simulink model "sampleModel7126_pp_1_1"  (R2018a)
settings: Solver=VariableStepAuto  StartTime=0.0  StopTime=10.0  RelTol=1e-3
undefined symbols (not defined in the file): DiscIntNeverNeededParam
libraries: simulink x367
(part 9 of 12)

== system sampleModel7126_pp_1_1/cfblk275/cfblk10 ==
  cfblk1 : Inport
  Action Port : ActionPort  ActionType=then
  cfblk10 : simulink/Continuous/PID Controller  Controller=PID  TimeDomain=Discrete-time  SampleTime=-1  IntegratorMethod=Forward Euler  FilterMethod=Forward Euler  Form=Parallel  UseFilter=on  ControllerParametersSource=internal  P=1  I=1  D=0  N=100  InitialConditionSource=internal  InitialConditionForIntegrator=0  InitialConditionForFilter=0  ExternalReset=none  LimitOutput=off  UpperSaturationLimit=inf  LowerSaturationLimit=-inf  LinearizeAsGain=off  AntiWindupMode=none  Kb=1  TrackingMode=off  Kt=1  PParamMin=[]  PParamMax=[]  IParamMin=[]  IParamMax=[]  DParamMin=[]  DParamMax=[]  NParamMin=[]  NParamMax=[]  KbParamMin=[]  KbParamMax=[]  KtParamMin=[]  KtParamMax=[]  POutMin=[]  POutMax=[]  IOutMin=[]  IOutMax=[]  DOutMin=[]  DOutMax=[]  NOutMin=[]  NOutMax=[]  KbOutMin=[]  KbOutMax=[]  KtOutMin=[]  KtOutMax=[]  IntegratorOutMin=[]  IntegratorOutMax=[]  FilterOutMin=[]  FilterOutMax=[]  SumOutMin=[]  SumOutMax=[]  SumI1OutMin=[]  SumI1OutMax=[]  SumI2OutMin=[]  SumI2OutMax=[]  SumI3OutMin=[]  SumI3OutMax=[]  SumDOutMin=[]  SumDOutMax=[]  SaturationOutMin=[]  SaturationOutMax=[]  IntegratorContinuousStateAttributes=''  IntegratorStateMustResolveToSignalObject=off  IntegratorRTWStateStorageClass=Auto  FilterContinuousStateAttributes=''  FilterStateMustResolveToSignalObject=off  FilterRTWStateStorageClass=Auto  DifferentiatorICPrevScaledInput=0  DifferentiatorOutMin=[]  DifferentiatorOutMax=[]  FilterDiffOutCoefMin=[]  FilterDiffOutCoefMax=[]  SumDenOutMin=[]  SumDenOutMax=[]  SumNumOutMin=[]  SumNumOutMax=[]  ReciprocalOutMin=[]  ReciprocalOutMax=[]  DivideOutMin=[]  DivideOutMax=[]  TunerSelectOption=Transfer Function Based (PID Tuner App)
  cfblk11 : DiscreteFilter
  cfblk12 : Delay  ShowEnablePort=on
      settings: InputPortMap=u0,e6
  cfblk13 : Delay
  cfblk3 : Subsystem  TreatAsAtomicUnit=on
  cfblk4 : Subsystem  TreatAsAtomicUnit=on
  cfblk5 : Subsystem  TreatAsAtomicUnit=on
  cfblk6 : DiscreteFilter
  cfblk7 : DiscreteFilter
  cfblk8 : Subsystem  TreatAsAtomicUnit=on
  cfblk9 : simulink/Discrete/Difference  ICPrevInput=0.0  OutMin=[]  OutMax=[]  OutDataTypeStr=double  OutputDataTypeScalingMode=double  OutDataType=fixdt(1, 16)  OutScaling=2^-10  DoSatur=off
  cyemi_{765..776} (12 alike) : DataTypeConversion  OutDataTypeStr=double
  emi_1205 : Subsystem  TreatAsAtomicUnit=on
  emi_{128,1207,1700,1939} (4 alike) : If  IfExpression=Inf <= u1  SampleTime=[1 0]
  emi_{129,1208,1701,1940} (4 alike) : DataTypeConversion  OutDataTypeStr=double
  emi_126 : Subsystem  TreatAsAtomicUnit=on
  emi_1698 : Subsystem  TreatAsAtomicUnit=on
  emi_1937 : Subsystem  TreatAsAtomicUnit=on
  cfblk2 : Outport
  wires:
  cfblk7/1 -> cfblk2/1, emi_1940/1
  cfblk11/1 -> cyemi_771/1, cyemi_775/1
  cyemi_765/1 -> cfblk10/1
  cfblk9/1 -> cyemi_765/1
  cyemi_766/1 -> cfblk11/1
  cfblk1/1 -> cyemi_766/1
  cyemi_767/1 -> cfblk12/1
  cfblk10/1 -> cyemi_767/1
  cyemi_768/1 -> cfblk12/2
  cfblk13/1 -> cyemi_768/1
  cyemi_769/1 -> cfblk13/1
  cfblk12/1 -> cyemi_772/1, emi_129/1
  cyemi_773/1 -> cfblk6/1
  cyemi_774/1 -> cfblk7/1
  cfblk6/1 -> cyemi_774/1, emi_1701/1
  cyemi_776/1 -> cfblk9/1
  cyemi_772/1 -> cfblk5/1(emi_124)
  cfblk5/1(emi_125) -> cyemi_769/1
  emi_128/1 -> cfblk5/Action
  emi_128/2 -> emi_126/Action
  emi_129/1 -> emi_128/1
  cyemi_775/1 -> cfblk8/1(emi_1203)
  cfblk8/1(emi_1204) -> cyemi_773/1
  emi_1207/1 -> cfblk8/Action
  emi_1207/2 -> emi_1205/Action
  emi_1208/1 -> emi_1207/1
  cyemi_770/1 -> cfblk3/1(emi_1696)
  cfblk3/1(emi_1697) -> emi_1208/1, cyemi_776/1
  emi_1700/1 -> cfblk3/Action
  emi_1700/2 -> emi_1698/Action
  emi_1701/1 -> emi_1700/1
  cyemi_771/1 -> cfblk4/1(emi_1935)
  cfblk4/1(emi_1936) -> cyemi_770/1
  emi_1939/1 -> cfblk4/Action
  emi_1939/2 -> emi_1937/Action
  emi_1940/1 -> emi_1939/1

== system sampleModel7126_pp_1_1/cfblk275/cfblk11 ==
  cfblk1 : Inport
  Action Port : ActionPort  ActionType=else
  cfblk10 : simulink/Discrete/Transfer Fcn Real Zero  ZeroZ=0.75  ICPrevInput=0.0  DoSatur=off
      settings: SourceProductName=Simulink  SourceProductBaseCode=SL
  cfblk11 : Subsystem  TreatAsAtomicUnit=on
  cfblk12 : DiscreteIntegrator  SampleTime=-1  OutDataTypeStr=double  ICPrevOutput=DiscIntNeverNeededParam  ICPrevScaledInput=DiscIntNeverNeededParam
  cfblk13 : DiscreteZeroPole  Poles=[0 0.5]  Gain=1  SampleTime=-1
  cfblk14 : Subsystem  TreatAsAtomicUnit=on
  cfblk18 : Delay
  cfblk3 : Subsystem  TreatAsAtomicUnit=on
  cfblk4 : simulink/Continuous/PID Controller  Controller=PID  TimeDomain=Discrete-time  SampleTime=-1  IntegratorMethod=Forward Euler  FilterMethod=Forward Euler  Form=Parallel  UseFilter=on  ControllerParametersSource=internal  P=1  I=1  D=0  N=100  InitialConditionSource=internal  InitialConditionForIntegrator=0  InitialConditionForFilter=0  ExternalReset=none  LimitOutput=off  UpperSaturationLimit=inf  LowerSaturationLimit=-inf  LinearizeAsGain=off  AntiWindupMode=none  Kb=1  TrackingMode=off  Kt=1  PParamMin=[]  PParamMax=[]  IParamMin=[]  IParamMax=[]  DParamMin=[]  DParamMax=[]  NParamMin=[]  NParamMax=[]  KbParamMin=[]  KbParamMax=[]  KtParamMin=[]  KtParamMax=[]  POutMin=[]  POutMax=[]  IOutMin=[]  IOutMax=[]  DOutMin=[]  DOutMax=[]  NOutMin=[]  NOutMax=[]  KbOutMin=[]  KbOutMax=[]  KtOutMin=[]  KtOutMax=[]  IntegratorOutMin=[]  IntegratorOutMax=[]  FilterOutMin=[]  FilterOutMax=[]  SumOutMin=[]  SumOutMax=[]  SumI1OutMin=[]  SumI1OutMax=[]  SumI2OutMin=[]  SumI2OutMax=[]  SumI3OutMin=[]  SumI3OutMax=[]  SumDOutMin=[]  SumDOutMax=[]  SaturationOutMin=[]  SaturationOutMax=[]  IntegratorContinuousStateAttributes=''  IntegratorStateMustResolveToSignalObject=off  IntegratorRTWStateStorageClass=Auto  FilterContinuousStateAttributes=''  FilterStateMustResolveToSignalObject=off  FilterRTWStateStorageClass=Auto  DifferentiatorICPrevScaledInput=0  DifferentiatorOutMin=[]  DifferentiatorOutMax=[]  FilterDiffOutCoefMin=[]  FilterDiffOutCoefMax=[]  SumDenOutMin=[]  SumDenOutMax=[]  SumNumOutMin=[]  SumNumOutMax=[]  ReciprocalOutMin=[]  ReciprocalOutMax=[]  DivideOutMin=[]  DivideOutMax=[]  TunerSelectOption=Transfer Function Based (PID Tuner App)
  cfblk5 : DiscreteZeroPole  Poles=[0 0.5]  Gain=1  SampleTime=-1
  cfblk6 : DiscreteStateSpace  SampleTime=-1
  cfblk7 : Delay  ShowEnablePort=on
      settings: InputPortMap=u0,e6
  cfblk8 : UnitDelay  SampleTime=-1
  cfblk9 : Subsystem  TreatAsAtomicUnit=on
  cyemi_{778..791} (14 alike) : DataTypeConversion  OutDataTypeStr=double
  emi_1322 : Subsystem  TreatAsAtomicUnit=on
  emi_{567,609,1324,2191} (4 alike) : If  IfExpression=0 <= u1  SampleTime=[1 0]
  emi_{568,610,1325,2192} (4 alike) : DataTypeConversion  OutDataTypeStr=double
  emi_2189 : Subsystem  TreatAsAtomicUnit=on
  emi_565 : Subsystem  TreatAsAtomicUnit=on
  emi_607 : Subsystem  TreatAsAtomicUnit=on
  cfblk2 : Outport
  cfblk15 : Outport  Port=2
  cfblk16 : Outport  Port=3
  cfblk17 : Outport  Port=4
  wires:
  cfblk5/1 -> cyemi_779/1, cyemi_780/1, emi_610/1
  cfblk8/1 -> cfblk15/1
  cfblk10/1 -> cfblk16/1, cyemi_784/1
  cfblk6/1 -> cfblk17/1, cyemi_790/1
  cyemi_778/1 -> cfblk10/1
  cfblk7/1 -> cyemi_778/1
  cyemi_780/1 -> cfblk12/1
  cyemi_781/1 -> cfblk13/1
  cfblk4/1 -> cyemi_782/1
  cyemi_783/1 -> cfblk18/1
  cyemi_785/1 -> cfblk4/1
  cfblk13/1 -> cyemi_785/1
  cyemi_786/1 -> cfblk5/1
  cfblk18/1 -> cyemi_786/1, emi_1325/1
  cyemi_787/1 -> cfblk6/1
  cyemi_788/1 -> cfblk7/1
  cfblk1/1 -> cyemi_788/1
  cyemi_789/1 -> cfblk7/2
  cfblk12/1 -> cyemi_789/1, emi_2192/1
  cyemi_790/1 -> cfblk8/1
  cyemi_782/1 -> cfblk14/1(emi_563)
  cfblk14/1(emi_564) -> cfblk2/1
  emi_567/1 -> cfblk14/Action
  emi_567/2 -> emi_565/Action
  emi_568/1 -> emi_567/1
  cyemi_784/1 -> cfblk3/1(emi_605)
  cfblk3/1(emi_606) -> cyemi_787/1
  emi_609/1 -> cfblk3/Action
  emi_609/2 -> emi_607/Action
  emi_610/1 -> emi_609/1
  cyemi_791/1 -> cfblk9/1(emi_1320)
  cfblk9/1(emi_1321) -> cyemi_783/1
  emi_1324/1 -> cfblk9/Action
  emi_1324/2 -> emi_1322/Action
  emi_1325/1 -> emi_1324/1
  cyemi_779/1 -> cfblk11/1(emi_2187)
  cfblk11/1(emi_2188) -> emi_568/1, cyemi_791/1, cyemi_781/1
  emi_2191/1 -> cfblk11/Action
  emi_2191/2 -> emi_2189/Action
  emi_2192/1 -> emi_2191/1

== system sampleModel7126_pp_1_1/cfblk276/cfblk14 ==
  emi_1820 : Inport
  Action Port : ActionPort  ActionType=then
  cfblk14 : Delay
  emi_1821 : Outport
  wires:
  emi_1820/1 -> cfblk14/1
  cfblk14/1 -> emi_1821/1

== system sampleModel7126_pp_1_1/cfblk276/cfblk3 ==
  emi_238 : Inport
  Action Port : ActionPort  ActionType=then
  cfblk3 : simulink/Discrete/Transfer Fcn First Order  PoleZ=0.95  ICPrevOutput=0.0  DoSatur=off
      settings: SourceProductName=Simulink
  emi_239 : Outport
  wires:
  emi_238/1 -> cfblk3/1
  cfblk3/1 -> emi_239/1

== system sampleModel7126_pp_1_1/cfblk276/cfblk4 ==
  emi_79 : Inport
  Action Port : ActionPort  ActionType=then
  cfblk4 : UnitDelay  SampleTime=-1
  emi_80 : Outport
  wires:
  emi_79/1 -> cfblk4/1
  cfblk4/1 -> emi_80/1

== system sampleModel7126_pp_1_1/cfblk276/cfblk5 ==
  emi_767 : Inport
  Action Port : ActionPort  ActionType=then
  cfblk5 : DiscreteZeroPole  Poles=[0 0.5]  Gain=1  SampleTime=-1
  emi_768 : Outport
  wires:
  emi_767/1 -> cfblk5/1
  cfblk5/1 -> emi_768/1

== system sampleModel7126_pp_1_1/cfblk276/cfblk6 ==
  emi_1102 : Inport
  emi_1103 : Inport  Port=2
  Action Port : ActionPort  ActionType=then
  cfblk6 : Delay  ShowEnablePort=on
      settings: InputPortMap=u0,e6
  emi_1104 : Outport
  wires:
  emi_1102/1 -> cfblk6/1
  emi_1103/1 -> cfblk6/2
  cfblk6/1 -> emi_1104/1

== system sampleModel7126_pp_1_1/cfblk276/cfblk7 ==
  emi_1355 : Inport
  Action Port : ActionPort  ActionType=then
  cfblk7 : Delay
  emi_1356 : Outport
  wires:
  emi_1355/1 -> cfblk7/1
  cfblk7/1 -> emi_1356/1

== system sampleModel7126_pp_1_1/cfblk276/emi_1105 ==
  Action Port : ActionPort  ActionType=else
  emi_1106 : Assertion

== system sampleModel7126_pp_1_1/cfblk276/emi_1357 ==
  Action Port : ActionPort  ActionType=else
  emi_1358 : Assertion

== system sampleModel7126_pp_1_1/cfblk276/emi_1822 ==
  Action Port : ActionPort  ActionType=else
  emi_1823 : Assertion

== system sampleModel7126_pp_1_1/cfblk276/emi_240 ==
  Action Port : ActionPort  ActionType=else
  emi_241 : Assertion

== system sampleModel7126_pp_1_1/cfblk276/emi_769 ==
  Action Port : ActionPort  ActionType=else
  emi_770 : Assertion

== system sampleModel7126_pp_1_1/cfblk276/emi_81 ==
  Action Port : ActionPort  ActionType=else
  emi_82 : Assertion

== system sampleModel7126_pp_1_1/cfblk277/cfblk11 ==
  emi_746 : Inport
  Action Port : ActionPort  ActionType=then
  cfblk11 : Delay
  emi_747 : Outport
  wires:
  emi_746/1 -> cfblk11/1
  cfblk11/1 -> emi_747/1

== system sampleModel7126_pp_1_1/cfblk277/cfblk13 ==
  emi_1639 : Inport
  Action Port : ActionPort  ActionType=then
  cfblk13 : simulink/Discrete/Transfer Fcn Lead or Lag  PoleZ=0.95  ZeroZ=0.75  ICPrevOutput=0.0  ICPrevInput=0.0  DoSatur=off
      settings: SourceProductName=Simulink  SourceProductBaseCode=SL
  emi_1640 : Outport
  wires:
  emi_1639/1 -> cfblk13/1
  cfblk13/1 -> emi_1640/1

== system sampleModel7126_pp_1_1/cfblk277/cfblk18 ==
  cfblk1 : Inport
  cfblk8 : Inport  Port=2
  Action Port : ActionPort  ActionType=then
  cfblk3 : Subsystem  TreatAsAtomicUnit=on
  cfblk4 : DiscreteFir
  cfblk5 : Subsystem  TreatAsAtomicUnit=on
  cfblk6 : DiscreteZeroPole  Poles=[0 0.5]  Gain=1  SampleTime=-1
  cfblk7 : Subsystem  TreatAsAtomicUnit=on
  cfblk9 : Delay
  cyemi_{823..829} (7 alike) : DataTypeConversion  OutDataTypeStr=double
  emi_2154 : Subsystem  TreatAsAtomicUnit=on
  emi_2156 : If  IfExpression=Inf <= u1  SampleTime=[1 0]
  emi_2157 : DataTypeConversion  OutDataTypeStr=double
  emi_551 : Subsystem  TreatAsAtomicUnit=on
  emi_553 : If  IfExpression=Inf <= u1
  emi_554 : DataTypeConversion  OutDataTypeStr=double
  emi_940 : Subsystem  TreatAsAtomicUnit=on
  emi_942 : If  IfExpression=Inf <= u1  SampleTime=[1 0]
  emi_943 : DataTypeConversion  OutDataTypeStr=double
  cfblk2 : Outport
  wires:
  cfblk6/1 -> cyemi_823/1
  cyemi_824/1 -> cfblk4/1
  cyemi_826/1 -> cfblk6/1
  cfblk8/1 -> cyemi_826/1
  cfblk9/1 -> cyemi_827/1, emi_943/1
  cfblk1/1 -> cyemi_828/1
  cyemi_829/1 -> cfblk9/1
  cfblk4/1 -> cyemi_829/1, emi_554/1, emi_2157/1
  cyemi_823/1 -> cfblk3/1(emi_549)
  cfblk3/1(emi_550) -> cfblk2/1
  emi_553/1 -> cfblk3/Action
  emi_553/2 -> emi_551/Action
  emi_554/1 -> emi_553/1
  cyemi_825/1 -> cfblk5/1(emi_938)
  cfblk5/1(emi_939) -> cyemi_824/1
  emi_942/1 -> cfblk5/Action
  emi_942/2 -> emi_940/Action
  emi_943/1 -> emi_942/1
  cyemi_827/1 -> cfblk7/1(emi_2151)
  cyemi_828/1 -> cfblk7/2(emi_2152)
  cfblk7/1(emi_2153) -> cyemi_825/1
  emi_2156/1 -> cfblk7/Action
  emi_2156/2 -> emi_2154/Action
  emi_2157/1 -> emi_2156/1

== system sampleModel7126_pp_1_1/cfblk277/cfblk19 ==
  cfblk1 : Inport
  Action Port : ActionPort  ActionType=else
  cfblk{9..12} (4 alike) : Delay
  cfblk3 : simulink/Continuous/PID Controller (2DOF)  Controller=PID  TimeDomain=Discrete-time  SampleTime=-1  IntegratorMethod=Forward Euler  FilterMethod=Forward Euler  Form=Parallel  UseFilter=on  ControllerParametersSource=internal  P=1  I=1  D=0  N=100  b=1  c=1  InitialConditionSource=internal  InitialConditionForIntegrator=0  InitialConditionForFilter=0  ExternalReset=none  LimitOutput=off  UpperSaturationLimit=inf  LowerSaturationLimit=-inf  LinearizeAsGain=off  AntiWindupMode=none  Kb=1  TrackingMode=off  Kt=1  PParamMin=[]  PParamMax=[]  IParamMin=[]  IParamMax=[]  DParamMin=[]  DParamMax=[]  NParamMin=[]  NParamMax=[]  bParamMin=[]  bParamMax=[]  cParamMin=[]  cParamMax=[]  KbParamMin=[]  KbParamMax=[]  KtParamMin=[]  KtParamMax=[]  POutMin=[]  POutMax=[]  IOutMin=[]  IOutMax=[]  DOutMin=[]  DOutMax=[]  NOutMin=[]  NOutMax=[]  bOutMin=[]  bOutMax=[]  cOutMin=[]  cOutMax=[]  KbOutMin=[]  KbOutMax=[]  KtOutMin=[]  KtOutMax=[]  IntegratorOutMin=[]  IntegratorOutMax=[]  FilterOutMin=[]  FilterOutMax=[]  SumOutMin=[]  SumOutMax=[]  Sum1OutMin=[]  Sum1OutMax=[]  Sum2OutMin=[]  Sum2OutMax=[]  Sum3OutMin=[]  Sum3OutMax=[]  SumI1OutMin=[]  SumI1OutMax=[]  SumI2OutMin=[]  SumI2OutMax=[]  SumI3OutMin=[]  SumI3OutMax=[]  SumDOutMin=[]  SumDOutMax=[]  SaturationOutMin=[]  SaturationOutMax=[]  IntegratorContinuousStateAttributes=''  IntegratorStateMustResolveToSignalObject=off  IntegratorRTWStateStorageClass=Auto  FilterContinuousStateAttributes=''  FilterStateMustResolveToSignalObject=off  FilterRTWStateStorageClass=Auto  DifferentiatorICPrevScaledInput=0  DifferentiatorOutMin=[]  DifferentiatorOutMax=[]  FilterDiffOutCoefMin=[]  FilterDiffOutCoefMax=[]  SumDenOutMin=[]  SumDenOutMax=[]  SumNumOutMin=[]  SumNumOutMax=[]  ReciprocalOutMin=[]  ReciprocalOutMax=[]  DivideOutMin=[]  DivideOutMax=[]  TunerSelectOption=Transfer Function Based (PID Tuner App)
  cfblk4 : Delay  ShowEnablePort=on
      settings: InputPortMap=u0,e6
  cfblk5 : Subsystem  TreatAsAtomicUnit=on
  cfblk6 : Subsystem  TreatAsAtomicUnit=on
  cfblk7 : Delay  ShowEnablePort=on
      settings: InputPortMap=u0,e6
  cfblk8 : Subsystem  TreatAsAtomicUnit=on
  cyemi_{831..843} (13 alike) : DataTypeConversion  OutDataTypeStr=double
  emi_1599 : Subsystem  TreatAsAtomicUnit=on
  emi_1601 : If  IfExpression=Inf <= u1  SampleTime=[1 0]
  emi_1602 : DataTypeConversion  OutDataTypeStr=double
  emi_1908 : Subsystem  TreatAsAtomicUnit=on
  emi_1910 : If  IfExpression=Inf <= u1  SampleTime=[1 0]
  emi_1911 : DataTypeConversion  OutDataTypeStr=double
  emi_381 : Subsystem  TreatAsAtomicUnit=on
  emi_383 : If  IfExpression=Inf <= u1  SampleTime=[1 0]
  emi_384 : DataTypeConversion  OutDataTypeStr=double
  cfblk2 : Outport
  wires:
  cfblk1/1 -> cfblk2/1
  cfblk4/1 -> cyemi_831/1, cyemi_843/1
  cfblk3/1 -> cyemi_836/1, cyemi_841/1
  cfblk7/1 -> cyemi_837/1, cyemi_842/1
  cyemi_831/1 -> cfblk10/1
  cyemi_832/1 -> cfblk11/1
  cyemi_833/1 -> cfblk12/1
  cyemi_834/1 -> cfblk3/1
  cfblk9/1 -> cyemi_834/1, emi_1911/1
  cyemi_835/1 -> cfblk3/2
  cfblk10/1 -> cyemi_835/1, emi_1602/1
  cyemi_836/1 -> cfblk4/1
  cyemi_837/1 -> cfblk4/2
  cfblk12/1 -> cyemi_838/1, emi_384/1
  cyemi_840/1 -> cfblk7/1
  cfblk11/1 -> cyemi_840/1
  cyemi_841/1 -> cfblk7/2
  cyemi_843/1 -> cfblk9/1
  cyemi_839/1 -> cfblk6/1(emi_379)
  cfblk6/1(emi_380) -> cyemi_833/1
  emi_383/1 -> cfblk6/Action
  emi_383/2 -> emi_381/Action
  emi_384/1 -> emi_383/1
  cyemi_842/1 -> cfblk8/1(emi_1597)
  cfblk8/1(emi_1598) -> cyemi_832/1
  emi_1601/1 -> cfblk8/Action
  emi_1601/2 -> emi_1599/Action
  emi_1602/1 -> emi_1601/1
  cyemi_838/1 -> cfblk5/1(emi_1906)
  cfblk5/1(emi_1907) -> cyemi_839/1
  emi_1910/1 -> cfblk5/Action
  emi_1910/2 -> emi_1908/Action
  emi_1911/1 -> emi_1910/1

== system sampleModel7126_pp_1_1/cfblk277/cfblk21 ==
  emi_1646 : Inport
  Action Port : ActionPort  ActionType=then
  cfblk21 : Delay
  emi_1647 : Outport
  wires:
  emi_1646/1 -> cfblk21/1
  cfblk21/1 -> emi_1647/1

== system sampleModel7126_pp_1_1/cfblk277/cfblk23 ==
  emi_2059 : Inport
  Action Port : ActionPort  ActionType=then
  cfblk23 : Delay
  emi_2060 : Outport
  wires:
  emi_2059/1 -> cfblk23/1
  cfblk23/1 -> emi_2060/1

== system sampleModel7126_pp_1_1/cfblk277/cfblk3 ==
  emi_1327 : Inport
  Action Port : ActionPort  ActionType=then
  cfblk3 : simulink/Discrete/Transfer Fcn Real Zero  ZeroZ=0.75  ICPrevInput=0.0  DoSatur=off
      settings: SourceProductName=Simulink  SourceProductBaseCode=SL
  emi_1328 : Outport
  wires:
  emi_1327/1 -> cfblk3/1
  cfblk3/1 -> emi_1328/1

== system sampleModel7126_pp_1_1/cfblk277/cfblk5 ==
  emi_2087 : Inport
  Action Port : ActionPort  ActionType=then
  cfblk5 : Delay
  emi_2088 : Outport
  wires:
  emi_2087/1 -> cfblk5/1
  cfblk5/1 -> emi_2088/1

== system sampleModel7126_pp_1_1/cfblk277/cfblk6 ==
  emi_1440 : Inport
  Action Port : ActionPort  ActionType=then
  cfblk6 : UnitDelay  SampleTime=-1
  emi_1441 : Outport
  wires:
  emi_1440/1 -> cfblk6/1
  cfblk6/1 -> emi_1441/1

== system sampleModel7126_pp_1_1/cfblk277/cfblk7 ==
  emi_626 : Inport
  Action Port : ActionPort  ActionType=then
  cfblk7 : UnitDelay  SampleTime=-1
  emi_627 : Outport
  wires:
  emi_626/1 -> cfblk7/1
  cfblk7/1 -> emi_627/1

== system sampleModel7126_pp_1_1/cfblk277/cfblk8 ==
  emi_216 : Inport
  Action Port : ActionPort  ActionType=then
  cfblk8 : DiscreteFilter
  emi_217 : Outport
  wires:
  emi_216/1 -> cfblk8/1
  cfblk8/1 -> emi_217/1

== system sampleModel7126_pp_1_1/cfblk277/emi_1329 ==
  Action Port : ActionPort  ActionType=else
  emi_1330 : Assertion

== system sampleModel7126_pp_1_1/cfblk277/emi_1442 ==
  Action Port : ActionPort  ActionType=else
  emi_1443 : Assertion

== system sampleModel7126_pp_1_1/cfblk277/emi_1641 ==
  Action Port : ActionPort  ActionType=else
  emi_1642 : Assertion

== system sampleModel7126_pp_1_1/cfblk277/emi_1648 ==
  Action Port : ActionPort  ActionType=else
  emi_1649 : Assertion

== system sampleModel7126_pp_1_1/cfblk277/emi_2061 ==
  Action Port : ActionPort  ActionType=else
  emi_2062 : Assertion

== system sampleModel7126_pp_1_1/cfblk277/emi_2089 ==
  Action Port : ActionPort  ActionType=else
  emi_2090 : Assertion

== system sampleModel7126_pp_1_1/cfblk277/emi_218 ==
  Action Port : ActionPort  ActionType=else
  emi_219 : Assertion

== system sampleModel7126_pp_1_1/cfblk277/emi_628 ==
  Action Port : ActionPort  ActionType=else
  emi_629 : Assertion

== system sampleModel7126_pp_1_1/cfblk277/emi_748 ==
  Action Port : ActionPort  ActionType=else
  emi_749 : Assertion

== system sampleModel7126_pp_1_1/cfblk278/cfblk12 ==
  cfblk1 : Inport
  Action Port : ActionPort  ActionType=then
  cfblk10 : DiscreteFir
  cfblk11 : simulink/Discrete/Transfer Fcn Lead or Lag  PoleZ=0.95  ZeroZ=0.75  ICPrevOutput=0.0  ICPrevInput=0.0  DoSatur=off
      settings: SourceProductName=Simulink  SourceProductBaseCode=SL
  cfblk12 : Subsystem  TreatAsAtomicUnit=on
  cfblk{4,13..15} (4 alike) : Delay
  cfblk3 : simulink/Discrete/Transfer Fcn Lead or Lag  PoleZ=0.95  ZeroZ=0.75  ICPrevOutput=0.0  ICPrevInput=0.0  DoSatur=off
      settings: SourceProductName=Simulink  SourceProductBaseCode=SL
  cfblk5 : simulink/Continuous/PID Controller  Controller=PID  TimeDomain=Discrete-time  SampleTime=-1  IntegratorMethod=Forward Euler  FilterMethod=Forward Euler  Form=Parallel  UseFilter=on  ControllerParametersSource=internal  P=1  I=1  D=0  N=100  InitialConditionSource=internal  InitialConditionForIntegrator=0  InitialConditionForFilter=0  ExternalReset=none  LimitOutput=off  UpperSaturationLimit=inf  LowerSaturationLimit=-inf  LinearizeAsGain=off  AntiWindupMode=none  Kb=1  TrackingMode=off  Kt=1  PParamMin=[]  PParamMax=[]  IParamMin=[]  IParamMax=[]  DParamMin=[]  DParamMax=[]  NParamMin=[]  NParamMax=[]  KbParamMin=[]  KbParamMax=[]  KtParamMin=[]  KtParamMax=[]  POutMin=[]  POutMax=[]  IOutMin=[]  IOutMax=[]  DOutMin=[]  DOutMax=[]  NOutMin=[]  NOutMax=[]  KbOutMin=[]  KbOutMax=[]  KtOutMin=[]  KtOutMax=[]  IntegratorOutMin=[]  IntegratorOutMax=[]  FilterOutMin=[]  FilterOutMax=[]  SumOutMin=[]  SumOutMax=[]  SumI1OutMin=[]  SumI1OutMax=[]  SumI2OutMin=[]  SumI2OutMax=[]  SumI3OutMin=[]  SumI3OutMax=[]  SumDOutMin=[]  SumDOutMax=[]  SaturationOutMin=[]  SaturationOutMax=[]  IntegratorContinuousStateAttributes=''  IntegratorStateMustResolveToSignalObject=off  IntegratorRTWStateStorageClass=Auto  FilterContinuousStateAttributes=''  FilterStateMustResolveToSignalObject=off  FilterRTWStateStorageClass=Auto  DifferentiatorICPrevScaledInput=0  DifferentiatorOutMin=[]  DifferentiatorOutMax=[]  FilterDiffOutCoefMin=[]  FilterDiffOutCoefMax=[]  SumDenOutMin=[]  SumDenOutMax=[]  SumNumOutMin=[]  SumNumOutMax=[]  ReciprocalOutMin=[]  ReciprocalOutMax=[]  DivideOutMin=[]  DivideOutMax=[]  TunerSelectOption=Transfer Function Based (PID Tuner App)
  cfblk6 : Subsystem  TreatAsAtomicUnit=on
  cfblk7 : DiscreteIntegrator  SampleTime=-1  OutDataTypeStr=double  ICPrevOutput=DiscIntNeverNeededParam  ICPrevScaledInput=DiscIntNeverNeededParam
  cfblk8 : simulink/Discrete/Tapped Delay  vinit=0.0  samptime=-1  NumDelays=1  DelayOrder=Oldest  includeCurrent=off
  cfblk9 : DiscreteFir
  cyemi_{859..871} (13 alike) : DataTypeConversion  OutDataTypeStr=double
  emi_2139 : Subsystem  TreatAsAtomicUnit=on
  emi_2141 : If  IfExpression=Inf <= u1  SampleTime=[1 0]
  emi_2142 : DataTypeConversion  OutDataTypeStr=double
  emi_74 : Subsystem  TreatAsAtomicUnit=on
  emi_76 : If  IfExpression=Inf <= u1  SampleTime=[1 0]
  emi_77 : DataTypeConversion  OutDataTypeStr=double
  cfblk2 : Outport
  wires:
  cfblk1/1 -> cfblk2/1
  cyemi_859/1 -> cfblk10/1
  cfblk9/1 -> cyemi_859/1, emi_2142/1
  cyemi_860/1 -> cfblk11/1
  cfblk8/1 -> cyemi_860/1
  cfblk7/1 -> cyemi_861/1
  cyemi_862/1 -> cfblk13/1
  cfblk11/1 -> cyemi_862/1
  cyemi_863/1 -> cfblk14/1
  cyemi_864/1 -> cfblk15/1
  cfblk10/1 -> cyemi_864/1
  cyemi_865/1 -> cfblk3/1
  cfblk13/1 -> cyemi_865/1
  cyemi_866/1 -> cfblk4/1
  cfblk14/1 -> cyemi_866/1
  cyemi_867/1 -> cfblk5/1
  cfblk15/1 -> cyemi_867/1
  cfblk4/1 -> cyemi_868/1
  cyemi_869/1 -> cfblk7/1
  cfblk5/1 -> cyemi_869/1
  cyemi_870/1 -> cfblk8/1
  cfblk3/1 -> cyemi_870/1
  cyemi_871/1 -> cfblk9/1
  cyemi_868/1 -> cfblk6/1(emi_72)
  cfblk6/1(emi_73) -> cyemi_863/1
  emi_76/1 -> cfblk6/Action
  emi_76/2 -> emi_74/Action
  emi_77/1 -> emi_76/1
  cyemi_861/1 -> cfblk12/1(emi_2137)
  cfblk12/1(emi_2138) -> emi_77/1, cyemi_871/1
  emi_2141/1 -> cfblk12/Action
  emi_2141/2 -> emi_2139/Action
  emi_2142/1 -> emi_2141/1

== system sampleModel7126_pp_1_1/cfblk278/cfblk13 ==
  cfblk1 : Inport
  cfblk8 : Inport  Port=2
  cfblk9 : Inport  Port=3
  Action Port : ActionPort  ActionType=else
  cfblk3 : DiscreteFir
  cfblk4 : Delay
  cfblk5 : simulink/Discrete/Transfer Fcn Real Zero  ZeroZ=0.75  ICPrevInput=0.0  DoSatur=off
      settings: SourceProductName=Simulink  SourceProductBaseCode=SL
  cfblk6 : DiscreteTransferFcn
  cfblk7 : DiscreteIntegrator  SampleTime=-1  OutDataTypeStr=double  ICPrevOutput=DiscIntNeverNeededParam  ICPrevScaledInput=DiscIntNeverNeededParam
  cyemi_{875..879} (5 alike) : DataTypeConversion  OutDataTypeStr=double
  cfblk2 : Outport
  wires:
  cfblk9/1 -> cfblk2/1
  cyemi_875/1 -> cfblk3/1
  cfblk1/1 -> cyemi_875/1
  cyemi_876/1 -> cfblk4/1
  cfblk3/1 -> cyemi_876/1
  cyemi_877/1 -> cfblk5/1
  cfblk7/1 -> cyemi_877/1
  cyemi_878/1 -> cfblk6/1
  cfblk5/1 -> cyemi_878/1
  cyemi_879/1 -> cfblk7/1
  cfblk8/1 -> cyemi_879/1

== system sampleModel7126_pp_1_1/cfblk278/cfblk14 ==
  cfblk1 : Inport
  cfblk9 : Inport  Port=2
  cfblk10 : Inport  Port=3
  cfblk11 : Inport  Port=4
  cfblk12 : Inport  Port=5
  cfblk13 : Inport  Port=6
  cfblk14 : Inport  Port=7
  cfblk15 : Inport  Port=8
  Action Port : ActionPort  ActionType=then
  cfblk17 : Delay
  cfblk3 : DiscreteFilter
  cfblk4 : Delay  DelayLengthSource=Input port
      settings: InputPortMap=u0,p1
  cfblk5 : DiscreteTransferFcn
  cfblk6 : Delay  DelayLengthSource=Input port
      settings: InputPortMap=u0,p1
  cfblk7 : DiscreteStateSpace  SampleTime=-1
  cfblk8 : UnitDelay  SampleTime=-1
  cyemi_{888..896} (9 alike) : DataTypeConversion  OutDataTypeStr=double
  cfblk2 : Outport
  cfblk16 : Outport  Port=2
  wires:
  cfblk11/1 -> cfblk16/1
  cfblk7/1 -> cfblk2/1
  cyemi_888/1 -> cfblk17/1
  cfblk8/1 -> cyemi_888/1
  cyemi_889/1 -> cfblk3/1
  cfblk5/1 -> cyemi_889/1
  cyemi_890/1 -> cfblk4/1
  cfblk9/1 -> cyemi_890/1
  cyemi_891/1 -> cfblk4/2
  cfblk1/1 -> cyemi_891/1
  cyemi_892/1 -> cfblk5/1
  cfblk15/1 -> cyemi_892/1
  cyemi_893/1 -> cfblk6/1
  cfblk3/1 -> cyemi_893/1
  cyemi_894/1 -> cfblk6/2
  cfblk17/1 -> cyemi_894/1
  cyemi_895/1 -> cfblk7/1
  cfblk12/1 -> cyemi_895/1
  cyemi_896/1 -> cfblk8/1
  cfblk6/1 -> cyemi_896/1

== system sampleModel7126_pp_1_1/cfblk278/cfblk15 ==
  cfblk1 : Inport
  cfblk13 : Inport  Port=2
  cfblk14 : Inport  Port=3
  cfblk15 : Inport  Port=4
  Action Port : ActionPort  ActionType=else
  cfblk10 : simulink/Discrete/Tapped Delay  vinit=0.0  samptime=-1  NumDelays=1  DelayOrder=Oldest  includeCurrent=off
  cfblk11 : UnitDelay  SampleTime=-1
  cfblk12 : DiscreteZeroPole  Poles=[0 0.5]  Gain=1  SampleTime=-1
  cfblk17 : Delay
  cfblk3 : simulink/Continuous/PID Controller (2DOF)  Controller=PID  TimeDomain=Discrete-time  SampleTime=-1  IntegratorMethod=Forward Euler  FilterMethod=Forward Euler  Form=Parallel  UseFilter=on  ControllerParametersSource=internal  P=1  I=1  D=0  N=100  b=1  c=1  InitialConditionSource=internal  InitialConditionForIntegrator=0  InitialConditionForFilter=0  ExternalReset=none  LimitOutput=off  UpperSaturationLimit=inf  LowerSaturationLimit=-inf  LinearizeAsGain=off  AntiWindupMode=none  Kb=1  TrackingMode=off  Kt=1  PParamMin=[]  PParamMax=[]  IParamMin=[]  IParamMax=[]  DParamMin=[]  DParamMax=[]  NParamMin=[]  NParamMax=[]  bParamMin=[]  bParamMax=[]  cParamMin=[]  cParamMax=[]  KbParamMin=[]  KbParamMax=[]  KtParamMin=[]  KtParamMax=[]  POutMin=[]  POutMax=[]  IOutMin=[]  IOutMax=[]  DOutMin=[]  DOutMax=[]  NOutMin=[]  NOutMax=[]  bOutMin=[]  bOutMax=[]  cOutMin=[]  cOutMax=[]  KbOutMin=[]  KbOutMax=[]  KtOutMin=[]  KtOutMax=[]  IntegratorOutMin=[]  IntegratorOutMax=[]  FilterOutMin=[]  FilterOutMax=[]  SumOutMin=[]  SumOutMax=[]  Sum1OutMin=[]  Sum1OutMax=[]  Sum2OutMin=[]  Sum2OutMax=[]  Sum3OutMin=[]  Sum3OutMax=[]  SumI1OutMin=[]  SumI1OutMax=[]  SumI2OutMin=[]  SumI2OutMax=[]  SumI3OutMin=[]  SumI3OutMax=[]  SumDOutMin=[]  SumDOutMax=[]  SaturationOutMin=[]  SaturationOutMax=[]  IntegratorContinuousStateAttributes=''  IntegratorStateMustResolveToSignalObject=off  IntegratorRTWStateStorageClass=Auto  FilterContinuousStateAttributes=''  FilterStateMustResolveToSignalObject=off  FilterRTWStateStorageClass=Auto  DifferentiatorICPrevScaledInput=0  DifferentiatorOutMin=[]  DifferentiatorOutMax=[]  FilterDiffOutCoefMin=[]  FilterDiffOutCoefMax=[]  SumDenOutMin=[]  SumDenOutMax=[]  SumNumOutMin=[]  SumNumOutMax=[]  ReciprocalOutMin=[]  ReciprocalOutMax=[]  DivideOutMin=[]  DivideOutMax=[]  TunerSelectOption=Transfer Function Based (PID Tuner App)
  cfblk4 : Subsystem  TreatAsAtomicUnit=on
  cfblk5 : simulink/Discrete/Transfer Fcn First Order  PoleZ=0.95  ICPrevOutput=0.0  DoSatur=off
      settings: SourceProductName=Simulink
  cfblk6 : Subsystem  TreatAsAtomicUnit=on
  cfblk7 : DiscreteIntegrator  SampleTime=-1  OutDataTypeStr=double  ICPrevOutput=DiscIntNeverNeededParam  ICPrevScaledInput=DiscIntNeverNeededParam
  cfblk8 : DiscreteZeroPole  Poles=[0 0.5]  Gain=1  SampleTime=-1
  cfblk9 : DiscreteIntegrator  SampleTime=-1  OutDataTypeStr=double  ICPrevOutput=DiscIntNeverNeededParam  ICPrevScaledInput=DiscIntNeverNeededParam
  cyemi_{901..912} (12 alike) : DataTypeConversion  OutDataTypeStr=double
  emi_469 : Subsystem  TreatAsAtomicUnit=on
  emi_471 : If  IfExpression=0 <= u1  SampleTime=[1 0]
  emi_472 : DataTypeConversion  OutDataTypeStr=double
  emi_657 : Subsystem  TreatAsAtomicUnit=on
  emi_659 : If  IfExpression=0 <= u1  SampleTime=[1 0]
  emi_660 : DataTypeConversion  OutDataTypeStr=double
  cfblk2 : Outport
  cfblk16 : Outport  Port=2
  wires:
  cfblk1/1 -> cfblk16/1
  cfblk12/1 -> cfblk2/1
  cyemi_901/1 -> cfblk10/1
  cfblk14/1 -> cyemi_901/1
  cyemi_902/1 -> cfblk11/1
  cfblk7/1 -> cyemi_902/1
  cyemi_903/1 -> cfblk12/1
  cfblk3/1 -> cyemi_903/1
  cyemi_904/1 -> cfblk17/1
  cfblk11/1 -> cyemi_904/1
  cyemi_905/1 -> cfblk3/1
  cyemi_906/1 -> cfblk3/2
  cfblk8/1 -> cyemi_906/1
  cfblk5/1 -> cyemi_907/1
  cyemi_908/1 -> cfblk5/1
  cfblk10/1 -> cyemi_908/1, emi_472/1
  cfblk9/1 -> cyemi_909/1
  cyemi_910/1 -> cfblk7/1
  cfblk17/1 -> cyemi_910/1, emi_660/1
  cyemi_911/1 -> cfblk8/1
  cfblk15/1 -> cyemi_911/1
  cyemi_912/1 -> cfblk9/1
  cyemi_909/1 -> cfblk6/1(emi_467)
  cfblk6/1(emi_468) -> cyemi_905/1
  emi_471/1 -> cfblk6/Action
  emi_471/2 -> emi_469/Action
  emi_472/1 -> emi_471/1
  cyemi_907/1 -> cfblk4/1(emi_655)
  cfblk4/1(emi_656) -> cyemi_912/1
  emi_659/1 -> cfblk4/Action
  emi_659/2 -> emi_657/Action
  emi_660/1 -> emi_659/1

== system sampleModel7126_pp_1_1/cfblk278/cfblk5 ==
  emi_1066 : Inport
  emi_1067 : Inport  Port=2
  Action Port : ActionPort  ActionType=then
  cfblk5 : Delay  DelayLengthSource=Input port
      settings: InputPortMap=u0,p1
  emi_1068 : Outport
  wires:
  emi_1066/1 -> cfblk5/1
  emi_1067/1 -> cfblk5/2
  cfblk5/1 -> emi_1068/1

== system sampleModel7126_pp_1_1/cfblk278/emi_1069 ==
  Action Port : ActionPort  ActionType=else
  emi_1070 : Assertion

== system sampleModel7126_pp_1_1/cfblk279/cfblk10 ==
  emi_1088 : Inport
  Action Port : ActionPort  ActionType=then
  cfblk10 : Delay
  emi_1089 : Outport
  wires:
  emi_1088/1 -> cfblk10/1
  cfblk10/1 -> emi_1089/1

== system sampleModel7126_pp_1_1/cfblk279/cfblk11 ==
  emi_683 : Inport
  Action Port : ActionPort  ActionType=then
  cfblk11 : Delay
  emi_684 : Outport
  wires:
  emi_683/1 -> cfblk11/1
  cfblk11/1 -> emi_684/1

== system sampleModel7126_pp_1_1/cfblk279/cfblk3 ==
  emi_1173 : Inport
  Action Port : ActionPort  ActionType=then
  cfblk3 : simulink/Discrete/Transfer Fcn First Order  PoleZ=0.95  ICPrevOutput=0.0  DoSatur=off
      settings: SourceProductName=Simulink
  emi_1174 : Outport
  wires:
  emi_1173/1 -> cfblk3/1
  cfblk3/1 -> emi_1174/1

== system sampleModel7126_pp_1_1/cfblk279/cfblk4 ==
  emi_1 : Inport
  Action Port : ActionPort  ActionType=then
  cfblk4 : simulink/Discrete/Tapped Delay  vinit=0.0  samptime=-1  NumDelays=1  DelayOrder=Oldest  includeCurrent=off
  emi_2 : Outport
  wires:
  emi_1/1 -> cfblk4/1
  cfblk4/1 -> emi_2/1

== system sampleModel7126_pp_1_1/cfblk279/cfblk7 ==
  emi_803 : Inport
  emi_804 : Inport  Port=2
  Action Port : ActionPort  ActionType=then
  cfblk7 : Delay  ShowEnablePort=on
      settings: InputPortMap=u0,e6
  emi_805 : Outport
  wires:
  emi_803/1 -> cfblk7/1
  emi_804/1 -> cfblk7/2
  cfblk7/1 -> emi_805/1

== system sampleModel7126_pp_1_1/cfblk279/emi_1090 ==
  Action Port : ActionPort  ActionType=else
  emi_1091 : Assertion

== system sampleModel7126_pp_1_1/cfblk279/emi_1175 ==
  Action Port : ActionPort  ActionType=else
  emi_1176 : Assertion

== system sampleModel7126_pp_1_1/cfblk279/emi_3 ==
  Action Port : ActionPort  ActionType=else
  emi_4 : Assertion

== system sampleModel7126_pp_1_1/cfblk279/emi_685 ==
  Action Port : ActionPort  ActionType=else
  emi_686 : Assertion

== system sampleModel7126_pp_1_1/cfblk279/emi_806 ==
  Action Port : ActionPort  ActionType=else
  emi_807 : Assertion

== system sampleModel7126_pp_1_1/cfblk280/cfblk13 ==
  cfblk1 : Inport
  Action Port : ActionPort  ActionType=then
  cfblk3 : DiscreteTransferFcn
  cfblk4 : DiscreteFilter
  cfblk5 : simulink/Discrete/Transfer Fcn First Order  PoleZ=0.95  ICPrevOutput=0.0  DoSatur=off
      settings: SourceProductName=Simulink
  cfblk6 : Delay  DelayLengthSource=Input port
      settings: InputPortMap=u0,p1
  cfblk7 : Subsystem  TreatAsAtomicUnit=on
  cfblk9 : Delay
  cyemi_{943..950} (8 alike) : DataTypeConversion  OutDataTypeStr=double
  emi_2009 : Subsystem  TreatAsAtomicUnit=on
  emi_2011 : If  IfExpression=Inf <= u1  SampleTime=[1 0]
  emi_2012 : DataTypeConversion  OutDataTypeStr=double
  cfblk2 : Outport
  cfblk8 : Outport  Port=2
  wires:
  cfblk1/1 -> cfblk8/1, cyemi_945/1
  cfblk5/1 -> cyemi_947/1, cyemi_949/1
  cfblk6/1 -> cfblk2/1, cyemi_943/1, emi_2012/1
  cyemi_943/1 -> cfblk3/1
  cyemi_944/1 -> cfblk4/1
  cyemi_945/1 -> cfblk5/1
  cyemi_946/1 -> cfblk6/1
  cfblk9/1 -> cyemi_946/1
  cyemi_947/1 -> cfblk6/2
  cfblk3/1 -> cyemi_948/1
  cyemi_950/1 -> cfblk9/1
  cfblk4/1 -> cyemi_950/1
  cyemi_948/1 -> cfblk7/1(emi_2006)
  cyemi_949/1 -> cfblk7/2(emi_2007)
  cfblk7/1(emi_2008) -> cyemi_944/1
  emi_2011/1 -> cfblk7/Action
  emi_2011/2 -> emi_2009/Action
  emi_2012/1 -> emi_2011/1

== system sampleModel7126_pp_1_1/cfblk280/cfblk14 ==
  cfblk1 : Inport
  cfblk8 : Inport  Port=2
  cfblk9 : Inport  Port=3
  Action Port : ActionPort  ActionType=else
  cfblk11 : DataTypeConversion  OutDataTypeStr=double
  cfblk3 : Delay
  cfblk4 : simulink/Continuous/PID Controller  Controller=PID  TimeDomain=Discrete-time  SampleTime=-1  IntegratorMethod=Forward Euler  FilterMethod=Forward Euler  Form=Parallel  UseFilter=on  ControllerParametersSource=internal  P=1  I=1  D=0  N=100  InitialConditionSource=internal  InitialConditionForIntegrator=0  InitialConditionForFilter=0  ExternalReset=none  LimitOutput=off  UpperSaturationLimit=inf  LowerSaturationLimit=-inf  LinearizeAsGain=off  AntiWindupMode=none  Kb=1  TrackingMode=off  Kt=1  PParamMin=[]  PParamMax=[]  IParamMin=[]  IParamMax=[]  DParamMin=[]  DParamMax=[]  NParamMin=[]  NParamMax=[]  KbParamMin=[]  KbParamMax=[]  KtParamMin=[]  KtParamMax=[]  POutMin=[]  POutMax=[]  IOutMin=[]  IOutMax=[]  DOutMin=[]  DOutMax=[]  NOutMin=[]  NOutMax=[]  KbOutMin=[]  KbOutMax=[]  KtOutMin=[]  KtOutMax=[]  IntegratorOutMin=[]  IntegratorOutMax=[]  FilterOutMin=[]  FilterOutMax=[]  SumOutMin=[]  SumOutMax=[]  SumI1OutMin=[]  SumI1OutMax=[]  SumI2OutMin=[]  SumI2OutMax=[]  SumI3OutMin=[]  SumI3OutMax=[]  SumDOutMin=[]  SumDOutMax=[]  SaturationOutMin=[]  SaturationOutMax=[]  IntegratorContinuousStateAttributes=''  IntegratorStateMustResolveToSignalObject=off  IntegratorRTWStateStorageClass=Auto  FilterContinuousStateAttributes=''  FilterStateMustResolveToSignalObject=off  FilterRTWStateStorageClass=Auto  DifferentiatorICPrevScaledInput=0  DifferentiatorOutMin=[]  DifferentiatorOutMax=[]  FilterDiffOutCoefMin=[]  FilterDiffOutCoefMax=[]  SumDenOutMin=[]  SumDenOutMax=[]  SumNumOutMin=[]  SumNumOutMax=[]  ReciprocalOutMin=[]  ReciprocalOutMax=[]  DivideOutMin=[]  DivideOutMax=[]  TunerSelectOption=Transfer Function Based (PID Tuner App)
  cfblk5 : DiscreteZeroPole  Poles=[0 0.5]  Gain=1  SampleTime=-1
  cfblk6 : Delay
  cfblk7 : DiscreteZeroPole  Poles=[0 0.5]  Gain=1  SampleTime=-1
  cyemi_954 : DataTypeConversion  OutDataTypeStr=uint8
  cyemi_955 : DataTypeConversion  OutDataTypeStr=fixdt('ufix8_E6')
  cyemi_{956..959} (4 alike) : DataTypeConversion  OutDataTypeStr=double
  cfblk2 : Outport
  cfblk10 : Outport  Port=2
  wires:
  cfblk4/1 -> cfblk10/1
  cfblk9/1 -> cfblk2/1
  cyemi_954/1 -> cfblk11/1
  cfblk1/1 -> cyemi_954/1
  cyemi_955/1 -> cfblk3/1
  cfblk8/1 -> cyemi_955/1
  cyemi_956/1 -> cfblk4/1
  cfblk5/1 -> cyemi_956/1
  cyemi_957/1 -> cfblk5/1
  cfblk6/1 -> cyemi_957/1
  cyemi_958/1 -> cfblk6/1
  cfblk7/1 -> cyemi_958/1
  cyemi_959/1 -> cfblk7/1
  cfblk11/1 -> cyemi_959/1

== system sampleModel7126_pp_1_1/cfblk280/cfblk16 ==
  emi_308 : Inport
  Action Port : ActionPort  ActionType=then
  cfblk16 : Delay
  emi_309 : Outport
  wires:
  emi_308/1 -> cfblk16/1
  cfblk16/1 -> emi_309/1

== system sampleModel7126_pp_1_1/cfblk280/cfblk4 ==
  emi_358 : Inport
  Action Port : ActionPort  ActionType=then
  cfblk4 : simulink/Discrete/Transfer Fcn Lead or Lag  PoleZ=0.95  ZeroZ=0.75  ICPrevOutput=0.0  ICPrevInput=0.0  DoSatur=off
      settings: SourceProductName=Simulink  SourceProductBaseCode=SL
  emi_359 : Outport
  wires:
  emi_358/1 -> cfblk4/1
  cfblk4/1 -> emi_359/1

== system sampleModel7126_pp_1_1/cfblk280/emi_310 ==
  Action Port : ActionPort  ActionType=else
  emi_311 : Assertion

== system sampleModel7126_pp_1_1/cfblk280/emi_360 ==
  Action Port : ActionPort  ActionType=else
  emi_361 : Assertion

== system sampleModel7126_pp_1_1/cfblk281/cfblk3 ==
  emi_138 : Inport
  Action Port : ActionPort  ActionType=then
  cfblk3 : simulink/Discrete/Transfer Fcn Real Zero  ZeroZ=0.75  ICPrevInput=0.0  DoSatur=off
      settings: SourceProductName=Simulink  SourceProductBaseCode=SL
  emi_139 : Outport
  wires:
  emi_138/1 -> cfblk3/1
  cfblk3/1 -> emi_139/1

== system sampleModel7126_pp_1_1/cfblk281/emi_140 ==
  Action Port : ActionPort  ActionType=else
  emi_141 : Assertion

== system sampleModel7126_pp_1_1/cfblk282/cfblk3 ==
  emi_1848 : Inport
  Action Port : ActionPort  ActionType=then
  cfblk3 : simulink/Discrete/Tapped Delay  vinit=0.0  samptime=-1  NumDelays=1  DelayOrder=Oldest  includeCurrent=off
  emi_1849 : Outport
  wires:
  emi_1848/1 -> cfblk3/1
  cfblk3/1 -> emi_1849/1

== system sampleModel7126_pp_1_1/cfblk282/cfblk4 ==
  emi_1017 : Inport
  Action Port : ActionPort  ActionType=then
  cfblk4 : DiscreteIntegrator  SampleTime=-1  OutDataTypeStr=double  ICPrevOutput=DiscIntNeverNeededParam  ICPrevScaledInput=DiscIntNeverNeededParam
  emi_1018 : Outport
  wires:
  emi_1017/1 -> cfblk4/1
  cfblk4/1 -> emi_1018/1

== system sampleModel7126_pp_1_1/cfblk282/cfblk5 ==
  emi_1920 : Inport
  emi_1921 : Inport  Port=2
  Action Port : ActionPort  ActionType=then
  cfblk5 : Delay  ShowEnablePort=on
      settings: InputPortMap=u0,e6
  emi_1922 : Outport
  wires:
  emi_1920/1 -> cfblk5/1
  emi_1921/1 -> cfblk5/2
  cfblk5/1 -> emi_1922/1

== system sampleModel7126_pp_1_1/cfblk282/cfblk7 ==
  emi_1525 : Inport
  Action Port : ActionPort  ActionType=then
  cfblk7 : simulink/Discrete/Tapped Delay  vinit=0.0  samptime=-1  NumDelays=1  DelayOrder=Oldest  includeCurrent=off
  emi_1526 : Outport
  wires:
  emi_1525/1 -> cfblk7/1
  cfblk7/1 -> emi_1526/1

== system sampleModel7126_pp_1_1/cfblk282/emi_1019 ==
  Action Port : ActionPort  ActionType=else
  emi_1020 : Assertion

== system sampleModel7126_pp_1_1/cfblk282/emi_1527 ==
  Action Port : ActionPort  ActionType=else
  emi_1528 : Assertion

== system sampleModel7126_pp_1_1/cfblk282/emi_1850 ==
  Action Port : ActionPort  ActionType=else
  emi_1851 : Assertion

== system sampleModel7126_pp_1_1/cfblk282/emi_1923 ==
  Action Port : ActionPort  ActionType=else
  emi_1924 : Assertion

== system sampleModel7126_pp_1_1/cfblk283/cfblk12 ==
  emi_173 : Inport
  Action Port : ActionPort  ActionType=then
  cfblk12 : DiscreteFir
  emi_174 : Outport
  wires:
  emi_173/1 -> cfblk12/1
  cfblk12/1 -> emi_174/1

== system sampleModel7126_pp_1_1/cfblk283/cfblk4 ==
  emi_1010 : Inport
  Action Port : ActionPort  ActionType=then
  cfblk4 : simulink/Discrete/Transfer Fcn Real Zero  ZeroZ=0.75  ICPrevInput=0.0  DoSatur=off
      settings: SourceProductName=Simulink  SourceProductBaseCode=SL
  emi_1011 : Outport
  wires:
  emi_1010/1 -> cfblk4/1
  cfblk4/1 -> emi_1011/1

== system sampleModel7126_pp_1_1/cfblk283/cfblk7 ==
  emi_1618 : Inport
  Action Port : ActionPort  ActionType=then
  cfblk7 : simulink/Discrete/Tapped Delay  vinit=0.0  samptime=-1  NumDelays=1  DelayOrder=Oldest  includeCurrent=off
  emi_1619 : Outport
  wires:
  emi_1618/1 -> cfblk7/1
  cfblk7/1 -> emi_1619/1

== system sampleModel7126_pp_1_1/cfblk283/cfblk9 ==
  emi_832 : Inport
  Action Port : ActionPort  ActionType=then
  cfblk9 : simulink/Discrete/Transfer Fcn Lead or Lag  PoleZ=0.95  ZeroZ=0.75  ICPrevOutput=0.0  ICPrevInput=0.0  DoSatur=off
      settings: SourceProductName=Simulink  SourceProductBaseCode=SL
  emi_833 : Outport
  wires:
  emi_832/1 -> cfblk9/1
  cfblk9/1 -> emi_833/1

== system sampleModel7126_pp_1_1/cfblk283/emi_1012 ==
  Action Port : ActionPort  ActionType=else
  emi_1013 : Assertion

== system sampleModel7126_pp_1_1/cfblk283/emi_1620 ==
  Action Port : ActionPort  ActionType=else
  emi_1621 : Assertion

== system sampleModel7126_pp_1_1/cfblk283/emi_175 ==
  Action Port : ActionPort  ActionType=else
  emi_176 : Assertion

== system sampleModel7126_pp_1_1/cfblk283/emi_834 ==
  Action Port : ActionPort  ActionType=else
  emi_835 : Assertion

== system sampleModel7126_pp_1_1/cfblk284/cfblk10 ==
  cfblk1 : Inport
  cfblk10 : Inport  Port=2
  cfblk11 : Inport  Port=3
  cfblk12 : Inport  Port=4
  Action Port : ActionPort  ActionType=then
  cfblk3 : Subsystem  TreatAsAtomicUnit=on
  cfblk4 : DiscreteFir
  cfblk5 : DiscreteFir
  cfblk6 : Subsystem  TreatAsAtomicUnit=on
  cfblk7 : UnitDelay  SampleTime=-1
  cfblk8 : simulink/Discrete/Transfer Fcn Real Zero  ZeroZ=0.75  ICPrevInput=0.0  DoSatur=off
      settings: SourceProductName=Simulink  SourceProductBaseCode=SL
  cfblk9 : simulink/Discrete/Tapped Delay  vinit=0.0  samptime=-1  NumDelays=1  DelayOrder=Oldest  includeCurrent=off
  cyemi_{1019..1025} (7 alike) : DataTypeConversion  OutDataTypeStr=double
  emi_1378 : Subsystem  TreatAsAtomicUnit=on
  emi_1380 : If  IfExpression=0 <= u1
  emi_1381 : DataTypeConversion  OutDataTypeStr=double
  emi_600 : Subsystem  TreatAsAtomicUnit=on
  emi_602 : If  IfExpression=0 <= u1  SampleTime=[1 0]
  emi_603 : DataTypeConversion  OutDataTypeStr=double
  cfblk2 : Outport
  cfblk13 : Outport  Port=2
  cfblk14 : Outport  Port=3
  cfblk15 : Outport  Port=4
  wires:
  cfblk1/1 -> cfblk2/1, cyemi_1020/1
  cfblk5/1 -> cfblk15/1
  cfblk11/1 -> cfblk13/1
  cfblk9/1 -> cyemi_1019/1
  cyemi_1020/1 -> cfblk4/1
  cyemi_1021/1 -> cfblk5/1
  cfblk8/1 -> cyemi_1021/1
  cfblk12/1 -> cyemi_1022/1
  cyemi_1023/1 -> cfblk7/1
  cfblk10/1 -> cyemi_1023/1
  cyemi_1024/1 -> cfblk8/1
  cyemi_1025/1 -> cfblk9/1
  cfblk7/1 -> cyemi_1025/1, emi_1381/1
  cyemi_1022/1 -> cfblk6/1(emi_598)
  cfblk6/1(emi_599) -> cyemi_1024/1
  emi_602/1 -> cfblk6/Action
  emi_602/2 -> emi_600/Action
  emi_603/1 -> emi_602/1
  cyemi_1019/1 -> cfblk3/1(emi_1376)
  cfblk3/1(emi_1377) -> emi_603/1, cfblk14/1
  emi_1380/1 -> cfblk3/Action
  emi_1380/2 -> emi_1378/Action
  emi_1381/1 -> emi_1380/1

== system sampleModel7126_pp_1_1/cfblk284/cfblk11 ==
  cfblk1 : Inport
  cfblk13 : Inport  Port=2
  cfblk14 : Inport  Port=3
  Action Port : ActionPort  ActionType=else
  cfblk10 : Subsystem  TreatAsAtomicUnit=on
  cfblk11 : Subsystem  TreatAsAtomicUnit=on
  cfblk12 : simulink/Continuous/PID Controller (2DOF)  Controller=PID  TimeDomain=Discrete-time  SampleTime=-1  IntegratorMethod=Forward Euler  FilterMethod=Forward Euler  Form=Parallel  UseFilter=on  ControllerParametersSource=internal  P=1  I=1  D=0  N=100  b=1  c=1  InitialConditionSource=internal  InitialConditionForIntegrator=0  InitialConditionForFilter=0  ExternalReset=none  LimitOutput=off  UpperSaturationLimit=inf  LowerSaturationLimit=-inf  LinearizeAsGain=off  AntiWindupMode=none  Kb=1  TrackingMode=off  Kt=1  PParamMin=[]  PParamMax=[]  IParamMin=[]  IParamMax=[]  DParamMin=[]  DParamMax=[]  NParamMin=[]  NParamMax=[]  bParamMin=[]  bParamMax=[]  cParamMin=[]  cParamMax=[]  KbParamMin=[]  KbParamMax=[]  KtParamMin=[]  KtParamMax=[]  POutMin=[]  POutMax=[]  IOutMin=[]  IOutMax=[]  DOutMin=[]  DOutMax=[]  NOutMin=[]  NOutMax=[]  bOutMin=[]  bOutMax=[]  cOutMin=[]  cOutMax=[]  KbOutMin=[]  KbOutMax=[]  KtOutMin=[]  KtOutMax=[]  IntegratorOutMin=[]  IntegratorOutMax=[]  FilterOutMin=[]  FilterOutMax=[]  SumOutMin=[]  SumOutMax=[]  Sum1OutMin=[]  Sum1OutMax=[]  Sum2OutMin=[]  Sum2OutMax=[]  Sum3OutMin=[]  Sum3OutMax=[]  SumI1OutMin=[]  SumI1OutMax=[]  SumI2OutMin=[]  SumI2OutMax=[]  SumI3OutMin=[]  SumI3OutMax=[]  SumDOutMin=[]  SumDOutMax=[]  SaturationOutMin=[]  SaturationOutMax=[]  IntegratorContinuousStateAttributes=''  IntegratorStateMustResolveToSignalObject=off  IntegratorRTWStateStorageClass=Auto  FilterContinuousStateAttributes=''  FilterStateMustResolveToSignalObject=off  FilterRTWStateStorageClass=Auto  DifferentiatorICPrevScaledInput=0  DifferentiatorOutMin=[]  DifferentiatorOutMax=[]  FilterDiffOutCoefMin=[]  FilterDiffOutCoefMax=[]  SumDenOutMin=[]  SumDenOutMax=[]  SumNumOutMin=[]  SumNumOutMax=[]  ReciprocalOutMin=[]  ReciprocalOutMax=[]  DivideOutMin=[]  DivideOutMax=[]  TunerSelectOption=Transfer Function Based (PID Tuner App)
  cfblk16 : Delay
  cfblk3 : simulink/Discrete/Difference  ICPrevInput=0.0  OutMin=[]  OutMax=[]  OutDataTypeStr=double  OutputDataTypeScalingMode=double  OutDataType=fixdt(1, 16)  OutScaling=2^-10  DoSatur=off
  cfblk4 : Subsystem  TreatAsAtomicUnit=on
  cfblk5 : Delay
  cfblk6 : DiscreteZeroPole  Poles=[0 0.5]  Gain=1  SampleTime=-1
  cfblk7 : Delay
  cfblk8 : Subsystem  TreatAsAtomicUnit=on
  cfblk9 : UnitDelay  SampleTime=-1
  cyemi_{1029..1042} (14 alike) : DataTypeConversion  OutDataTypeStr=double
  emi_1464 : Subsystem  TreatAsAtomicUnit=on
  emi_1466 : If  IfExpression=0 <= u1  SampleTime=[1 0]
  emi_{487,1467,1588,1616} (4 alike) : DataTypeConversion  OutDataTypeStr=double
  emi_1585 : Subsystem  TreatAsAtomicUnit=on
  emi_1587 : If  IfExpression=0 <= u1  SampleTime=[1 0]
  emi_1613 : Subsystem  TreatAsAtomicUnit=on
  emi_1615 : If  IfExpression=0 <= u1  SampleTime=[1 0]
  emi_484 : Subsystem  TreatAsAtomicUnit=on
  emi_486 : If  IfExpression=0 <= u1
  cfblk2 : Outport
  cfblk15 : Outport  Port=2
  wires:
  cfblk1/1 -> cyemi_1033/1, cyemi_1040/1
  cfblk5/1 -> cfblk2/1, emi_1588/1
  cfblk16/1 -> cyemi_1029/1, emi_1467/1
  cfblk9/1 -> cyemi_1031/1, emi_1616/1
  cyemi_1032/1 -> cfblk12/1
  cfblk7/1 -> cyemi_1032/1
  cyemi_1033/1 -> cfblk12/2
  cyemi_1034/1 -> cfblk16/1
  cfblk3/1 -> cyemi_1034/1
  cyemi_1035/1 -> cfblk3/1
  cyemi_1037/1 -> cfblk5/1
  cfblk12/1 -> cyemi_1037/1
  cyemi_1038/1 -> cfblk6/1
  cfblk13/1 -> cyemi_1038/1
  cyemi_1039/1 -> cfblk7/1
  cfblk14/1 -> cyemi_1041/1
  cyemi_1042/1 -> cfblk9/1
  cfblk6/1 -> cyemi_1042/1, emi_487/1
  cyemi_1029/1 -> cfblk10/1(emi_481)
  cyemi_1030/1 -> cfblk10/2(emi_482)
  cfblk10/1(emi_483) -> cyemi_1035/1
  emi_486/1 -> cfblk10/Action
  emi_486/2 -> emi_484/Action
  emi_487/1 -> emi_486/1
  cyemi_1040/1 -> cfblk8/1(emi_1461)
  cyemi_1041/1 -> cfblk8/2(emi_1462)
  cfblk8/1(emi_1463) -> cyemi_1036/1
  emi_1466/1 -> cfblk8/Action
  emi_1466/2 -> emi_1464/Action
  emi_1467/1 -> emi_1466/1
  cyemi_1031/1 -> cfblk11/1(emi_1583)
  cfblk11/1(emi_1584) -> cfblk15/1
  emi_1587/1 -> cfblk11/Action
  emi_1587/2 -> emi_1585/Action
  emi_1588/1 -> emi_1587/1
  cyemi_1036/1 -> cfblk4/1(emi_1611)
  cfblk4/1(emi_1612) -> cyemi_1039/1, cyemi_1030/1
  emi_1615/1 -> cfblk4/Action
  emi_1615/2 -> emi_1613/Action
  emi_1616/1 -> emi_1615/1

== system sampleModel7126_pp_1_1/cfblk284/cfblk12 ==
  emi_1217 : Inport
  Action Port : ActionPort  ActionType=then
  cfblk12 : Delay
  emi_1218 : Outport
  wires:
  emi_1217/1 -> cfblk12/1
  cfblk12/1 -> emi_1218/1

== system sampleModel7126_pp_1_1/cfblk284/cfblk15 ==
  emi_1999 : Inport
  Action Port : ActionPort  ActionType=then
  cfblk15 : Delay
  emi_2000 : Outport
  wires:
  emi_1999/1 -> cfblk15/1
  cfblk15/1 -> emi_2000/1

== system sampleModel7126_pp_1_1/cfblk284/cfblk3 ==
  emi_1653 : Inport
  Action Port : ActionPort  ActionType=then
  cfblk3 : simulink/Discrete/Transfer Fcn Lead or Lag  PoleZ=0.95  ZeroZ=0.75  ICPrevOutput=0.0  ICPrevInput=0.0  DoSatur=off
      settings: SourceProductName=Simulink  SourceProductBaseCode=SL
  emi_1654 : Outport
  wires:
  emi_1653/1 -> cfblk3/1
  cfblk3/1 -> emi_1654/1

== system sampleModel7126_pp_1_1/cfblk284/emi_1219 ==
  Action Port : ActionPort  ActionType=else
  emi_1220 : Assertion

== system sampleModel7126_pp_1_1/cfblk284/emi_1655 ==
  Action Port : ActionPort  ActionType=else
  emi_1656 : Assertion

== system sampleModel7126_pp_1_1/cfblk284/emi_2001 ==
  Action Port : ActionPort  ActionType=else
  emi_2002 : Assertion

== system sampleModel7126_pp_1_1/cfblk285/cfblk6 ==
  emi_760 : Inport
  Action Port : ActionPort  ActionType=then
  cfblk6 : DiscreteZeroPole  Poles=[0 0.5]  Gain=1  SampleTime=-1
  emi_761 : Outport
  wires:
  emi_760/1 -> cfblk6/1
  cfblk6/1 -> emi_761/1

== system sampleModel7126_pp_1_1/cfblk285/emi_762 ==
  Action Port : ActionPort  ActionType=else
  emi_763 : Assertion

== system sampleModel7126_pp_1_1/cfblk286/cfblk5 ==
  emi_732 : Inport
  Action Port : ActionPort  ActionType=then
  cfblk5 : UnitDelay  SampleTime=-1
  emi_733 : Outport
  wires:
  emi_732/1 -> cfblk5/1
  cfblk5/1 -> emi_733/1

== system sampleModel7126_pp_1_1/cfblk286/emi_734 ==
  Action Port : ActionPort  ActionType=else
  emi_735 : Assertion
